simulink model "DC_Motor_Simulink"  (R2025b)
settings: Solver=ode45  StartTime=0.0  StopTime=5  RelTol=1e-3
settings Model: Creator=adesh  LastModifiedBy=adesh

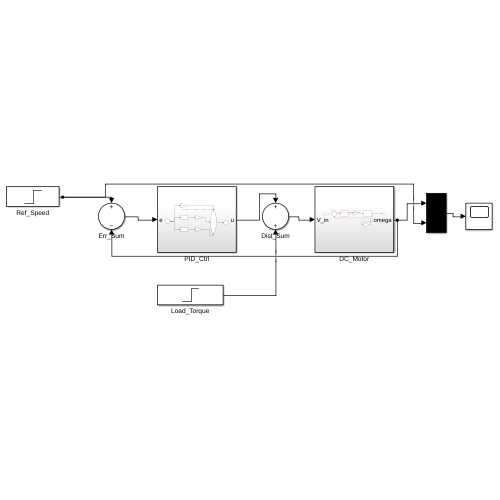
[thumbnail: Simulink's stored preview of the top-level diagram]
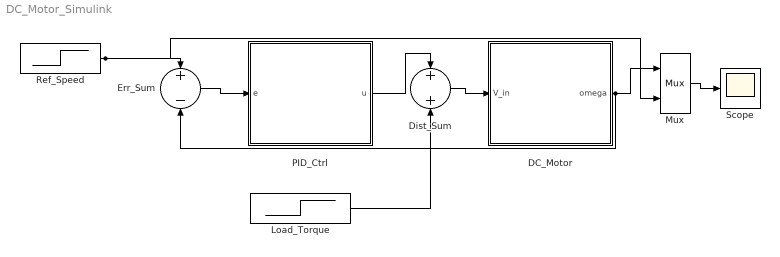
== system DC_Motor_Simulink ==
  DC_Motor : Subsystem
  Dist_Sum : Sum
  Err_Sum : Sum  Inputs=+-
  Load_Torque : Step  Time=2  After=0.5  SampleTime=0
  Mux : Mux  Inputs=2
  PID_Ctrl : Subsystem
  Ref_Speed : Step  Time=0  After=100  SampleTime=0
  Scope : Scope
  wires:
  Ref_Speed/1 -> Err_Sum/1, Mux/2
  DC_Motor/1(omega) -> Err_Sum/2, Mux/1
  Err_Sum/1 -> PID_Ctrl/1(e)
  PID_Ctrl/1(u) -> Dist_Sum/1
  Load_Torque/1 -> Dist_Sum/2
  Dist_Sum/1 -> DC_Motor/1(V_in)
  Mux/1 -> Scope/1

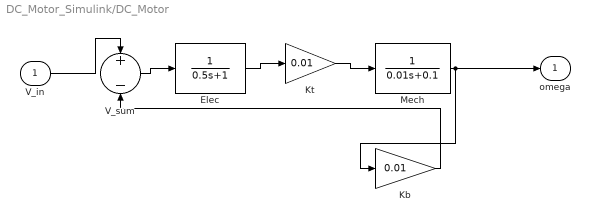
== system DC_Motor_Simulink/DC_Motor ==
  V_in : Inport
  Elec : TransferFcn  Denominator=[0.5 1]
  Kb : Gain  Gain=0.01
  Kt : Gain  Gain=0.01
  Mech : TransferFcn  Denominator=[0.01 0.1]
  V_sum : Sum  Inputs=+-
  omega : Outport
  wires:
  ? -> ?
  V_in/1 -> V_sum/1
  Kb/1 -> V_sum/2
  V_sum/1 -> Elec/1
  Elec/1 -> Kt/1
  Kt/1 -> Mech/1
  Mech/1 -> omega/1, Kb/1

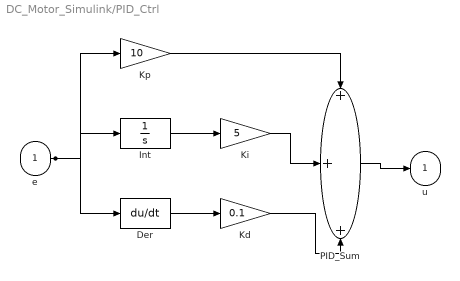
== system DC_Motor_Simulink/PID_Ctrl ==
  e : Inport
  Der : Derivative
  Int : Integrator
  Kd : Gain  Gain=0.1
  Ki : Gain  Gain=5
  Kp : Gain  Gain=10
  PID_Sum : Sum  Inputs=+++
  u : Outport
  wires:
  ? -> ?
  e/1 -> Kp/1, Int/1, Der/1
  Int/1 -> Ki/1
  Der/1 -> Kd/1
  Kp/1 -> PID_Sum/1
  Ki/1 -> PID_Sum/2
  Kd/1 -> PID_Sum/3
  PID_Sum/1 -> u/1
